simulink model "exemplul2"  (Simulink 7.2)
settings: Solver=ode45  StartTime=0.0  StopTime=10.0  RelTol=1e-3
settings Model: Creator=Student  LastModifiedBy=Student

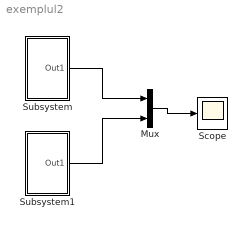
== system exemplul2 ==
  Mux : Mux  Inputs=2
  Scope : Scope
  Subsystem : Subsystem
  Subsystem1 : Subsystem
  wires:
  Mux/1 -> Scope/1
  Subsystem/1(Out1) -> Mux/1
  Subsystem1/1(Out1) -> Mux/2

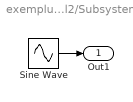
== system exemplul2/Subsystem ==
  Sine Wave : Sin  SampleTime=0
  Out1 : Outport
  wires:
  Sine Wave/1 -> Out1/1

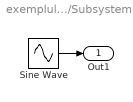
== system exemplul2/Subsystem1 ==
  Sine Wave : Sin  Frequency=2  SampleTime=0
  Out1 : Outport
  wires:
  Sine Wave/1 -> Out1/1
